simulink model "halfbridge"  (R2016a)
settings: Solver=ode2  StartTime=0.0  StopTime=0.1  FixedStep=1e-6  RelTol=1e-3
libraries: dspsigops x1
settings Model: Creator=Heath  LastModifiedBy=rtw141
settings DataIOCC: LimitDataPoints=on  SaveFormat=Array  SignalLoggingSaveFormat=ModelDataLogs  SignalLoggingName=sigsOut
settings OptimizationCC: ExpressionDepthLimit=2147483647
settings DebuggingCC: SaveWithParameterizedLinksMsg=none  UnderspecifiedInitializationDetection=Classic  MergeDetectMultiDrivingBlocksExec=none  SignalResolutionControl=TryResolveAllWithWarning  MultiTaskDSMMsg=warning  MultiTaskCondExecSysMsg=none  FcnCallInpInsideContextMsg=UseLocalSettings  StateNameClashWarn=warning
settings HardwareCC: ProdBitPerPointer=32  ProdLargestAtomicFloat=None  ProdIntDivRoundTo=Undefined  ProdEndianess=Unspecified  ProdWordSize=32  ProdHWDeviceType=32-bit Generic  TargetUnknown=on
settings ModelReferenceCC: PropagateSignalLabelsOutOfModel=off
settings GRTTargetCC: CombineOutputUpdateFcns=off  GRTInterface=on
settings ConfigComp: CovModelRefEnable=Off

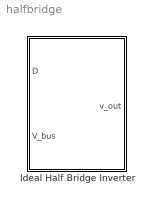
== system halfbridge ==
  "Ideal Half Bridge Inverter " : Subsystem

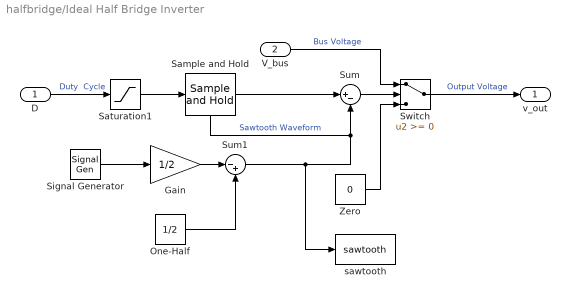
== system halfbridge/Ideal Half Bridge Inverter  ==
  D : Inport
  V_bus : Inport  Port=2
  Gain : Gain  Gain=1/2  SaturateOnIntegerOverflow=on  OutDataTypeStr=Inherit: Same as input  ParamDataTypeStr=Inherit: Same as input
  One-Half : Constant  Value=1/2
  Sample and Hold : dspsigops/Sample and Hold  trig=Falling edge  initCond=0  latchinput=off
  Saturation1 : Saturate  UpperLimit=1  LowerLimit=0
  Signal Generator : SignalGenerator  WaveForm=sawtooth  Frequency=10e3
  Sum : Sum  Inputs=|+-  SaturateOnIntegerOverflow=on
  Sum1 : Sum  Inputs=|-+  SaturateOnIntegerOverflow=on
  Switch : Switch  SaturateOnIntegerOverflow=on
  Zero : Constant  Value=0
  sawtooth : ToWorkspace  VariableName=sawtooth  SampleTime=-1
  v_out : Outport
  wires:
  Sum1/1 -> Sample and Hold/Trigger, Sum/2, sawtooth/1  "Sawtooth Waveform"
  Sum/1 -> Switch/2
  Zero/1 -> Switch/3
  V_bus/1 -> Switch/1  "Bus Voltage"
  Switch/1 -> v_out/1  "Output Voltage"
  Signal Generator/1 -> Gain/1
  Gain/1 -> Sum1/1
  One-Half/1 -> Sum1/2
  D/1 -> Saturation1/1  "Duty  Cycle"
  Sample and Hold/1 -> Sum/1
  Saturation1/1 -> Sample and Hold/1
